simulink library "PTCL_lib"  (Simulink 7.5)
settings: Solver=ode45  StartTime=0.0  StopTime=10.0  RelTol=1e-3
values from neighbouring files (symbols this model uses):
  pPTCL_kw_DeltaTMAvlPwr_TAB = Simulink.Parameter    [PTCL_par.m]
  pPTCL_kw_MaxIDeltaTMAvlPwr_C = Simulink.Parameter    [PTCL_par.m]
  pPTCL_kw_MaxPIDeltaTMAvlPwr_C = Simulink.Parameter    [PTCL_par.m]
  pPTCL_kw_MinIDeltaTMAvlPwr_C = Simulink.Parameter    [PTCL_par.m]
  pPTCL_kw_MinPIDeltaTMAvlPwr_C = Simulink.Parameter    [PTCL_par.m]
  pPTCL_kw_MinTMAvailPwr_C = Simulink.Parameter    [PTCL_par.m]
  pPTCL_kw_PIActDeltaPwrThrsh_C = Simulink.Parameter    [PTCL_par.m]
  pPTCL_kw_PIActHysterDeltaPwr_C = Simulink.Parameter    [PTCL_par.m]
  pPTCL_Nm_MaxTrq_CUR = Simulink.Parameter    [PTCL_par.m]
  pPTCL_Nmps_DrvTrqLowrRateLim_C = Simulink.Parameter    [PTCL_par.m]
  pPTCL_Nmps_DrvTrqUpprRateLim_C = Simulink.Parameter    [PTCL_par.m]
  pPTCL_Nmps_RcpTrqLowrRateLim_C = Simulink.Parameter    [PTCL_par.m]
  pPTCL_Nmps_RcpTrqUpprRateLim_C = Simulink.Parameter    [PTCL_par.m]
  pPTCL_pct_DrvEffiFac_C = Simulink.Parameter    [PTCL_par.m]
  pPTCL_pct_Mot1EffLowrLim_C = Simulink.Parameter    [PTCL_par.m]
  pPTCL_pct_Mot1EffUpprLim_C = Simulink.Parameter    [PTCL_par.m]
  pPTCL_pct_RcpEffiFac_C = Simulink.Parameter    [PTCL_par.m]
  pPTCL_ratio_KI4DeltaTMAvlPwr_CUR = Simulink.Parameter    [PTCL_par.m]
  pPTCL_ratio_KP4DeltaTMAvlPwr_CUR = Simulink.Parameter    [PTCL_par.m]
  pPTCL_ratio_KwToW_M = Simulink.Parameter    [PTCL_par.m]
  pPTCL_ratio_MotSpdFiltFac_C = Simulink.Parameter    [PTCL_par.m]
  pPTCL_ratio_PwrToTrqFac_M = Simulink.Parameter    [PTCL_par.m]
  pPTCL_ratio_WToKw_M = Simulink.Parameter    [PTCL_par.m]
  pPTCL_rpm_RevLowrLim_C = Simulink.Parameter    [PTCL_par.m]
  pPTCL_rpm_RevUpprLim_C = Simulink.Parameter    [PTCL_par.m]
  pPTCL_rpm_TMSpd_TAB = Simulink.Parameter    [PTCL_par.m]
undefined symbols (not defined in the file or in its folder): p_single_Minus_M, p_single_Zero_M, pESPI_kmph_MinSpdSnsrThd_C, pMCI_m_TireDiam_C, pMCI_ratio_KmPerHrToMtrPerSec_C, pMCI_ratio_TrsmRat_C, pMCI_s_NoOfSec_C
libraries: BaseOperationLib_Browser x114, simulink x1
(part 2 of 2)

== system PTCL_lib/PTCL/Algo/MCU1TrqLimCalc/EMSpdFlt ==
  rpm_MCU1TMSpd : Inport
  Abs2 : BaseOperationLib_Browser/Math Operations Changed/Abs  OutMax=[]  OutDataType=fixdt(1, 16)  OutScaling=2^0
  Integrator1 : UnitDelay  SampleTime=-1
      mask Display: patch([0 1 1 1 .75], [1 1 0 .75 1], [0 1 0]);
  LowPassTs : Constant  Value=pPTCL_ratio_MotSpdFiltFac_C
      mask Display: patch([0 1 1 1 .75], [1 1 0 .75 1], [0 1 0]);
  Saturation4 : BaseOperationLib_Browser/Discontinuities Unchanged/Saturation  UpperLimit=14000  LowerLimit=0.5  OutMin=[]  OutMax=[]  OutDataType=fixdt(1, 16)  OutScaling=2^0
      settings: AttributesFormatString=ULim:%<UpperLimit>\nLLim:%<LowerLimit>
  WerghtingFilter : BaseOperationLib_Browser/Discontinuities Unchanged/WerghtingFilter  SystemSampleTime=-1
  rpm_TMSpdFlt : Outport
  wires:
  Saturation4/1 -> rpm_TMSpdFlt/1
  Abs2/1 -> Saturation4/1
  rpm_MCU1TMSpd/1 -> WerghtingFilter/1
  WerghtingFilter/1 -> Abs2/1, Integrator1/1
  Integrator1/1 -> WerghtingFilter/2
  LowPassTs/1 -> WerghtingFilter/3

== system PTCL_lib/PTCL/Algo/MCU2TrqLimCalc/EMSpdFlt ==
  rpm_MCU2TMSpd : Inport
  Abs2 : BaseOperationLib_Browser/Math Operations Changed/Abs  OutMax=[]  OutDataType=fixdt(1, 16)  OutScaling=2^0
  Integrator1 : UnitDelay  SampleTime=-1
      mask Display: patch([0 1 1 1 .75], [1 1 0 .75 1], [0 1 0]);
  LowPassTs : Constant  Value=pPTCL_ratio_MotSpdFiltFac_C
      mask Display: patch([0 1 1 1 .75], [1 1 0 .75 1], [0 1 0]);
  Saturation4 : BaseOperationLib_Browser/Discontinuities Unchanged/Saturation  UpperLimit=14000  LowerLimit=0.5  OutMin=[]  OutMax=[]  OutDataType=fixdt(1, 16)  OutScaling=2^0
      settings: AttributesFormatString=ULim:%<UpperLimit>\nLLim:%<LowerLimit>
  WerghtingFilter : BaseOperationLib_Browser/Discontinuities Unchanged/WerghtingFilter  SystemSampleTime=-1
  rpm_TMSpdFlt : Outport
  wires:
  LowPassTs/1 -> WerghtingFilter/3
  Integrator1/1 -> WerghtingFilter/2
  WerghtingFilter/1 -> Integrator1/1, Abs2/1
  rpm_MCU2TMSpd/1 -> WerghtingFilter/1
  Abs2/1 -> Saturation4/1
  Saturation4/1 -> rpm_TMSpdFlt/1

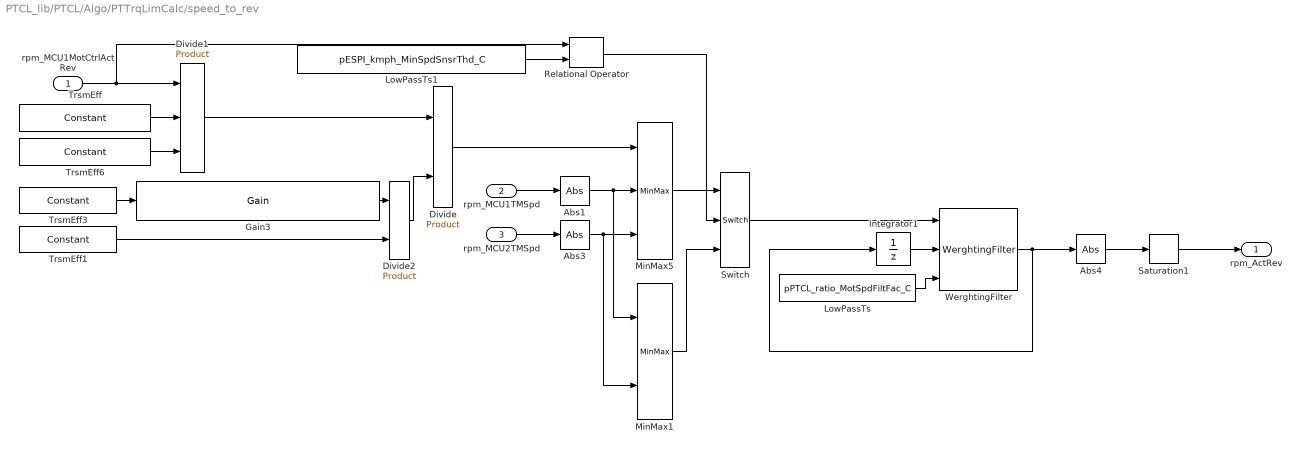
== system PTCL_lib/PTCL/Algo/PTTrqLimCalc/speed_to_rev ==
  rpm_MCU1MotCtrlActRev : Inport
  rpm_MCU1TMSpd : Inport  Port=2
  rpm_MCU2TMSpd : Inport  Port=3
  Abs1 : BaseOperationLib_Browser/Math Operations Changed/Abs  OutMax=[]  OutDataType=fixdt(1, 16)  OutScaling=2^0
  Abs3 : BaseOperationLib_Browser/Math Operations Changed/Abs  OutMax=[]  OutDataType=fixdt(1, 16)  OutScaling=2^0
  Abs4 : BaseOperationLib_Browser/Math Operations Changed/Abs  OutMax=[]  OutDataType=fixdt(1, 16)  OutScaling=2^0
  Divide : BaseOperationLib_Browser/Math Operations Changed/Product  Inputs=*/  Multiplication=Element-wise(.*)  OutMin=[]  OutMax=[]  OutDataType=fixdt(1,16,0)  OutScaling=[]
  Divide1 : BaseOperationLib_Browser/Math Operations Changed/Product  Inputs=***  Multiplication=Element-wise(.*)  OutMin=[]  OutMax=[]  OutDataType=fixdt(1,16,0)  OutScaling=[]
  Divide2 : BaseOperationLib_Browser/Math Operations Changed/Product  Inputs=**  Multiplication=Element-wise(.*)  OutMin=[]  OutMax=[]  OutDataType=fixdt(1,16,0)  OutScaling=[]
  Gain3 : BaseOperationLib_Browser/Math Operations Changed/Gain  Gain=pMCI_ratio_KmPerHrToMtrPerSec_C  Multiplication=Element-wise(K.*u)  ParamMin=[]  ParamMax=[]  ParameterDataType=fixdt(1, 16)  ParameterScalingMode=Best Precision: Matrix-wise  ParameterScaling=2^0  OutMin=[]  OutMax=[]  OutDataType=fixdt(1, 16)  OutScaling=2^0
  Integrator1 : UnitDelay  SampleTime=-1
      mask Display: patch([0 1 1 1 .75], [1 1 0 .75 1], [0 1 0]);
  LowPassTs : Constant  Value=pPTCL_ratio_MotSpdFiltFac_C
      mask Display: patch([0 1 1 1 .75], [1 1 0 .75 1], [0 1 0]);
  LowPassTs1 : Constant  Value=pESPI_kmph_MinSpdSnsrThd_C
      mask Display: patch([0 1 1 1 .75], [1 1 0 .75 1], [0 1 0]);
  MinMax1 : BaseOperationLib_Browser/Math Operations Changed/MinMax  Function=min  Inputs=2  InputSameDT=on  OutMin=[]  OutMax=[]  OutDataType=fixdt(1, 16)  OutScaling=2^0  SaturateOnIntegerOverflow=on
  MinMax5 : BaseOperationLib_Browser/Math Operations Changed/MinMax  Function=min  Inputs=3  InputSameDT=on  OutMin=[]  OutMax=[]  OutDataType=fixdt(1, 16)  OutScaling=2^0  SaturateOnIntegerOverflow=on
  Relational Operator : BaseOperationLib_Browser/Logic Operations Changed/Relational Operator  Operator=>=  InputSameDT=on  LogicOutDataTypeMode=Specify via dialog  LogicDataType=PDT_Bool  OutDataTypeStr=PDT_Bool
  Saturation1 : BaseOperationLib_Browser/Discontinuities Unchanged/Saturation  UpperLimit=pPTCL_rpm_RevUpprLim_C  LowerLimit=pPTCL_rpm_RevLowrLim_C  OutMin=[]  OutMax=[]  OutDataType=fixdt(1, 16)  OutScaling=2^0
      settings: AttributesFormatString=ULim:%<UpperLimit>\nLLim:%<LowerLimit>
  Switch : BaseOperationLib_Browser/Signal Routing Changed/Switch  Criteria=u2 ~= 0  Threshold=1  InputSameDT=on  OutMin=[]  OutMax=[]  OutDataType=fixdt(1,16,0)  OutScaling=[]  SaturateOnIntegerOverflow=on
  TrsmEff : BaseOperationLib_Browser/Sources&Sinks/Constant  Value=pMCI_ratio_TrsmRat_C  OutMin=[]  OutMax=[]  OutDataTypeMode=single  OutDataType=fixdt(1, 16)  ConRadixGroup=Use specified scaling  OutScaling=2^0  OutDataTypeStr=single
  TrsmEff1 : BaseOperationLib_Browser/Sources&Sinks/Constant  Value=pMCI_m_TireDiam_C  OutMin=[]  OutMax=[]  OutDataTypeMode=single  OutDataType=fixdt(1, 16)  ConRadixGroup=Use specified scaling  OutScaling=2^0  OutDataTypeStr=single
  TrsmEff3 : BaseOperationLib_Browser/Sources&Sinks/Constant  Value=pi  OutMin=[]  OutMax=[]  OutDataTypeMode=single  OutDataType=fixdt(1, 16)  ConRadixGroup=Use specified scaling  OutScaling=2^0  OutDataTypeStr=single
  TrsmEff6 : BaseOperationLib_Browser/Sources&Sinks/Constant  Value=pMCI_s_NoOfSec_C  OutMin=[]  OutMax=[]  OutDataTypeMode=single  OutDataType=fixdt(1, 16)  ConRadixGroup=Use specified scaling  OutScaling=2^0  OutDataTypeStr=single
  WerghtingFilter : BaseOperationLib_Browser/Discontinuities Unchanged/WerghtingFilter  SystemSampleTime=-1
  rpm_ActRev : Outport
  wires:
  TrsmEff1/1 -> Divide2/2
  rpm_MCU1MotCtrlActRev/1 -> Divide1/1, Relational Operator/1
  TrsmEff/1 -> Divide1/2
  TrsmEff3/1 -> Gain3/1
  Gain3/1 -> Divide2/1
  Divide1/1 -> Divide/1
  Divide2/1 -> Divide/2
  Switch/1 -> WerghtingFilter/1
  WerghtingFilter/1 -> Integrator1/1, Abs4/1
  Integrator1/1 -> WerghtingFilter/2
  LowPassTs/1 -> WerghtingFilter/3
  Divide/1 -> MinMax5/1
  rpm_MCU1TMSpd/1 -> Abs1/1
  rpm_MCU2TMSpd/1 -> Abs3/1
  MinMax1/1 -> Switch/3
  MinMax5/1 -> Switch/1
  LowPassTs1/1 -> Relational Operator/2
  Relational Operator/1 -> Switch/2
  Abs1/1 -> MinMax5/2, MinMax1/1
  Abs3/1 -> MinMax5/3, MinMax1/2
  Abs4/1 -> Saturation1/1
  Saturation1/1 -> rpm_ActRev/1
  TrsmEff6/1 -> Divide1/3

== system PTCL_lib/PTCL/Algo/CmptPwrLimCalc/BatMaxContiChrgPwrCalc/PwrCtrl ==
  ActPwr : Inport
  TgtPwr : Inport  Port=2
  Enable : EnablePort  StatesWhenEnabling=reset
  Abs1 : Abs  SaturateOnIntegerOverflow=on
      mask Display: patch([0 1 1 1 .75], [1 1 0 .75 1], [0 1 0]);
  Add2 : Sum  SaturateOnIntegerOverflow=on  InputSameDT=on  OutDataTypeStr=Inherit: Same as first input
      mask Display: patch([0 1 1 1 .75], [1 1 0 .75 1], [0 1 0]);
  Add5 : Sum  SaturateOnIntegerOverflow=on  InputSameDT=on  OutDataTypeStr=Inherit: Same as first input
      mask Display: patch([0 1 1 1 .75], [1 1 0 .75 1], [0 1 0]);
  Add6 : Sum  Inputs=+-  SaturateOnIntegerOverflow=on  InputSameDT=on  OutDataTypeStr=Inherit: Same as first input
      mask Display: patch([0 1 1 1 .75], [1 1 0 .75 1], [0 1 0]);
  Constant11 : Constant  Value=pPTCL_kw_MinIDeltaTMAvlPwr_C
      mask Display: patch([0 1 1 1 .75], [1 1 0 .75 1], [0 1 0]);
  Constant12 : Constant  Value=pPTCL_kw_MaxIDeltaTMAvlPwr_C  VectorParams1D=off
      mask Display: patch([0 1 1 1 .75], [1 1 0 .75 1], [0 1 0]);
  Constant13 : Constant  Value=pPTCL_kw_MinPIDeltaTMAvlPwr_C
      mask Display: patch([0 1 1 1 .75], [1 1 0 .75 1], [0 1 0]);
  Constant14 : Constant  Value=pPTCL_kw_MaxPIDeltaTMAvlPwr_C
      mask Display: patch([0 1 1 1 .75], [1 1 0 .75 1], [0 1 0]);
  Constant4 : Constant  Value=p_single_Zero_M
      mask Display: patch([0 1 1 1 .75], [1 1 0 .75 1], [0 1 0]);
  Lookup Table1 : BaseOperationLib_Browser/Lookup Tables Changed/Lookup Table  InputValues=pPTCL_kw_DeltaTMAvlPwr_TAB  Table=pPTCL_ratio_KP4DeltaTMAvlPwr_CUR  LookUpMeth=Interpolation-Use End Values  OutMin=[]  OutMax=[]  OutDataType=fixdt(1, 16)  OutScaling=2^0  OutDataTypeStr=Inherit: Inherit via back propagation  SaturateOnIntegerOverflow=on
      settings: AttributesFormatString=X:%<InputValues>\nTAB:%<Table>
  Lookup Table2 : BaseOperationLib_Browser/Lookup Tables Changed/Lookup Table  InputValues=pPTCL_kw_DeltaTMAvlPwr_TAB  Table=pPTCL_ratio_KI4DeltaTMAvlPwr_CUR  LookUpMeth=Interpolation-Use End Values  OutMin=[]  OutMax=[]  OutDataType=fixdt(1, 16)  OutScaling=2^0  OutDataTypeStr=Inherit: Inherit via back propagation  SaturateOnIntegerOverflow=on
      settings: AttributesFormatString=X:%<InputValues>\nTAB:%<Table>
  MinMax : BaseOperationLib_Browser/Math Operations Changed/MinMax  Function=min  Inputs=2  InputSameDT=on  OutMin=[]  OutMax=[]  OutDataType=fixdt(1,16,0)  OutScaling=[]  SaturateOnIntegerOverflow=on
  Product : BaseOperationLib_Browser/Math Operations Changed/Product  Inputs=2  Multiplication=Element-wise(.*)  OutMin=[]  OutMax=[]  OutDataType=fixdt(1,16,0)  OutScaling=[]  OutDataTypeStr=Inherit: Inherit via back propagation  RndMeth=Zero  SaturateOnIntegerOverflow=on
  Product1 : BaseOperationLib_Browser/Math Operations Changed/Product  Inputs=2  Multiplication=Element-wise(.*)  OutMin=[]  OutMax=[]  OutDataType=fixdt(1,16,0)  OutScaling=[]  OutDataTypeStr=Inherit: Inherit via back propagation  RndMeth=Zero  SaturateOnIntegerOverflow=on
  Saturation Dynamic1 : BaseOperationLib_Browser/Discontinuities Unchanged/Saturation Dynamic  SystemSampleTime=-1  OutMin=[]  OutMax=[]  OutDataTypeStr=Inherit: Same as second input  OutDataType=fixdt(1, 16)  OutScaling=2^-10  DoSatur=on
  Saturation Dynamic2 : BaseOperationLib_Browser/Discontinuities Unchanged/Saturation Dynamic  SystemSampleTime=-1  OutMin=[]  OutMax=[]  OutDataTypeStr=Inherit: Same as second input  OutDataType=fixdt(1, 16)  OutScaling=2^-10  DoSatur=on
  Signal Conversion : SignalConversion  ConversionOutput=Contiguous copy
  Unit Delay2 : BaseOperationLib_Browser/Discrete Unchanged /Unit Delay  X0=0  SampleTime=-1
  DeltaEMAvlPwr : Outport
  wires:
  ActPwr/1 -> Add6/2
  TgtPwr/1 -> Add6/1
  Add6/1 -> Product1/2, Product/2, Lookup Table2/1, Lookup Table1/1
  Add2/1 -> Saturation Dynamic2/2
  Constant14/1 -> Saturation Dynamic2/1
  Constant13/1 -> Saturation Dynamic2/3
  Product1/1 -> Add2/1
  Lookup Table1/1 -> Product1/1
  Product/1 -> Add5/1
  Lookup Table2/1 -> Product/1
  Saturation Dynamic1/1 -> Unit Delay2/1, Add2/2
  Add5/1 -> Saturation Dynamic1/2
  Constant12/1 -> Saturation Dynamic1/1
  Constant11/1 -> Saturation Dynamic1/3
  Unit Delay2/1 -> Add5/2
  Signal Conversion/1 -> DeltaEMAvlPwr/1
  Constant4/1 -> MinMax/1
  Saturation Dynamic2/1 -> MinMax/2
  MinMax/1 -> Abs1/1
  Abs1/1 -> Signal Conversion/1

== system PTCL_lib/PTCL/Algo/CmptPwrLimCalc/BatMaxContiDschPwrCalc/PwrCtrl ==
  ActPwr : Inport
  TgtPwr : Inport  Port=2
  Enable : EnablePort  StatesWhenEnabling=reset
  Abs1 : Abs  SaturateOnIntegerOverflow=on
      mask Display: patch([0 1 1 1 .75], [1 1 0 .75 1], [0 1 0]);
  Add2 : Sum  SaturateOnIntegerOverflow=on  InputSameDT=on  OutDataTypeStr=Inherit: Same as first input
      mask Display: patch([0 1 1 1 .75], [1 1 0 .75 1], [0 1 0]);
  Add5 : Sum  SaturateOnIntegerOverflow=on  InputSameDT=on  OutDataTypeStr=Inherit: Same as first input
      mask Display: patch([0 1 1 1 .75], [1 1 0 .75 1], [0 1 0]);
  Add6 : Sum  Inputs=+-  SaturateOnIntegerOverflow=on  InputSameDT=on  OutDataTypeStr=Inherit: Same as first input
      mask Display: patch([0 1 1 1 .75], [1 1 0 .75 1], [0 1 0]);
  Constant11 : Constant  Value=pPTCL_kw_MinIDeltaTMAvlPwr_C
      mask Display: patch([0 1 1 1 .75], [1 1 0 .75 1], [0 1 0]);
  Constant12 : Constant  Value=pPTCL_kw_MaxIDeltaTMAvlPwr_C  VectorParams1D=off
      mask Display: patch([0 1 1 1 .75], [1 1 0 .75 1], [0 1 0]);
  Constant13 : Constant  Value=pPTCL_kw_MinPIDeltaTMAvlPwr_C
      mask Display: patch([0 1 1 1 .75], [1 1 0 .75 1], [0 1 0]);
  Constant14 : Constant  Value=pPTCL_kw_MaxPIDeltaTMAvlPwr_C
      mask Display: patch([0 1 1 1 .75], [1 1 0 .75 1], [0 1 0]);
  Constant4 : Constant  Value=p_single_Zero_M
      mask Display: patch([0 1 1 1 .75], [1 1 0 .75 1], [0 1 0]);
  Lookup Table1 : BaseOperationLib_Browser/Lookup Tables Changed/Lookup Table  InputValues=pPTCL_kw_DeltaTMAvlPwr_TAB  Table=pPTCL_ratio_KP4DeltaTMAvlPwr_CUR  LookUpMeth=Interpolation-Use End Values  OutMin=[]  OutMax=[]  OutDataType=fixdt(1, 16)  OutScaling=2^0  OutDataTypeStr=Inherit: Inherit via back propagation  SaturateOnIntegerOverflow=on
      settings: AttributesFormatString=X:%<InputValues>\nTAB:%<Table>
  Lookup Table2 : BaseOperationLib_Browser/Lookup Tables Changed/Lookup Table  InputValues=pPTCL_kw_DeltaTMAvlPwr_TAB  Table=pPTCL_ratio_KI4DeltaTMAvlPwr_CUR  LookUpMeth=Interpolation-Use End Values  OutMin=[]  OutMax=[]  OutDataType=fixdt(1, 16)  OutScaling=2^0  OutDataTypeStr=Inherit: Inherit via back propagation  SaturateOnIntegerOverflow=on
      settings: AttributesFormatString=X:%<InputValues>\nTAB:%<Table>
  MinMax : BaseOperationLib_Browser/Math Operations Changed/MinMax  Function=min  Inputs=2  InputSameDT=on  OutMin=[]  OutMax=[]  OutDataType=fixdt(1,16,0)  OutScaling=[]  SaturateOnIntegerOverflow=on
  Product : BaseOperationLib_Browser/Math Operations Changed/Product  Inputs=2  Multiplication=Element-wise(.*)  OutMin=[]  OutMax=[]  OutDataType=fixdt(1,16,0)  OutScaling=[]  OutDataTypeStr=Inherit: Inherit via back propagation  RndMeth=Zero  SaturateOnIntegerOverflow=on
  Product1 : BaseOperationLib_Browser/Math Operations Changed/Product  Inputs=2  Multiplication=Element-wise(.*)  OutMin=[]  OutMax=[]  OutDataType=fixdt(1,16,0)  OutScaling=[]  OutDataTypeStr=Inherit: Inherit via back propagation  RndMeth=Zero  SaturateOnIntegerOverflow=on
  Saturation Dynamic1 : BaseOperationLib_Browser/Discontinuities Unchanged/Saturation Dynamic  SystemSampleTime=-1  OutMin=[]  OutMax=[]  OutDataTypeStr=Inherit: Same as second input  OutDataType=fixdt(1, 16)  OutScaling=2^-10  DoSatur=on
  Saturation Dynamic2 : BaseOperationLib_Browser/Discontinuities Unchanged/Saturation Dynamic  SystemSampleTime=-1  OutMin=[]  OutMax=[]  OutDataTypeStr=Inherit: Same as second input  OutDataType=fixdt(1, 16)  OutScaling=2^-10  DoSatur=on
  Signal Conversion : SignalConversion  ConversionOutput=Contiguous copy
  Unit Delay2 : BaseOperationLib_Browser/Discrete Unchanged /Unit Delay  X0=0  SampleTime=-1
  DeltaEMAvlPwr : Outport
  wires:
  ActPwr/1 -> Add6/2
  TgtPwr/1 -> Add6/1
  Add6/1 -> Product1/2, Product/2, Lookup Table2/1, Lookup Table1/1
  Add2/1 -> Saturation Dynamic2/2
  Constant14/1 -> Saturation Dynamic2/1
  Constant13/1 -> Saturation Dynamic2/3
  Product1/1 -> Add2/1
  Lookup Table1/1 -> Product1/1
  Product/1 -> Add5/1
  Lookup Table2/1 -> Product/1
  Saturation Dynamic1/1 -> Unit Delay2/1, Add2/2
  Add5/1 -> Saturation Dynamic1/2
  Constant12/1 -> Saturation Dynamic1/1
  Constant11/1 -> Saturation Dynamic1/3
  Unit Delay2/1 -> Add5/2
  Signal Conversion/1 -> DeltaEMAvlPwr/1
  Constant4/1 -> MinMax/1
  Saturation Dynamic2/1 -> MinMax/2
  MinMax/1 -> Abs1/1
  Abs1/1 -> Signal Conversion/1

== system PTCL_lib/PTCL/Algo/CmptPwrLimCalc/BatMaxPeakChrgPwrCalc/PwrCtrl ==
  ActPwr : Inport
  TgtPwr : Inport  Port=2
  Enable : EnablePort  StatesWhenEnabling=reset
  Abs1 : Abs  SaturateOnIntegerOverflow=on
      mask Display: patch([0 1 1 1 .75], [1 1 0 .75 1], [0 1 0]);
  Add2 : Sum  SaturateOnIntegerOverflow=on  InputSameDT=on  OutDataTypeStr=Inherit: Same as first input
      mask Display: patch([0 1 1 1 .75], [1 1 0 .75 1], [0 1 0]);
  Add5 : Sum  SaturateOnIntegerOverflow=on  InputSameDT=on  OutDataTypeStr=Inherit: Same as first input
      mask Display: patch([0 1 1 1 .75], [1 1 0 .75 1], [0 1 0]);
  Add6 : Sum  Inputs=+-  SaturateOnIntegerOverflow=on  InputSameDT=on  OutDataTypeStr=Inherit: Same as first input
      mask Display: patch([0 1 1 1 .75], [1 1 0 .75 1], [0 1 0]);
  Constant11 : Constant  Value=pPTCL_kw_MinIDeltaTMAvlPwr_C
      mask Display: patch([0 1 1 1 .75], [1 1 0 .75 1], [0 1 0]);
  Constant12 : Constant  Value=pPTCL_kw_MaxIDeltaTMAvlPwr_C  VectorParams1D=off
      mask Display: patch([0 1 1 1 .75], [1 1 0 .75 1], [0 1 0]);
  Constant13 : Constant  Value=pPTCL_kw_MinPIDeltaTMAvlPwr_C
      mask Display: patch([0 1 1 1 .75], [1 1 0 .75 1], [0 1 0]);
  Constant14 : Constant  Value=pPTCL_kw_MaxPIDeltaTMAvlPwr_C
      mask Display: patch([0 1 1 1 .75], [1 1 0 .75 1], [0 1 0]);
  Constant4 : Constant  Value=p_single_Zero_M
      mask Display: patch([0 1 1 1 .75], [1 1 0 .75 1], [0 1 0]);
  Lookup Table1 : BaseOperationLib_Browser/Lookup Tables Changed/Lookup Table  InputValues=pPTCL_kw_DeltaTMAvlPwr_TAB  Table=pPTCL_ratio_KP4DeltaTMAvlPwr_CUR  LookUpMeth=Interpolation-Use End Values  OutMin=[]  OutMax=[]  OutDataType=fixdt(1, 16)  OutScaling=2^0  OutDataTypeStr=Inherit: Inherit via back propagation  SaturateOnIntegerOverflow=on
      settings: AttributesFormatString=X:%<InputValues>\nTAB:%<Table>
  Lookup Table2 : BaseOperationLib_Browser/Lookup Tables Changed/Lookup Table  InputValues=pPTCL_kw_DeltaTMAvlPwr_TAB  Table=pPTCL_ratio_KI4DeltaTMAvlPwr_CUR  LookUpMeth=Interpolation-Use End Values  OutMin=[]  OutMax=[]  OutDataType=fixdt(1, 16)  OutScaling=2^0  OutDataTypeStr=Inherit: Inherit via back propagation  SaturateOnIntegerOverflow=on
      settings: AttributesFormatString=X:%<InputValues>\nTAB:%<Table>
  MinMax : BaseOperationLib_Browser/Math Operations Changed/MinMax  Function=min  Inputs=2  InputSameDT=on  OutMin=[]  OutMax=[]  OutDataType=fixdt(1,16,0)  OutScaling=[]  SaturateOnIntegerOverflow=on
  Product : BaseOperationLib_Browser/Math Operations Changed/Product  Inputs=2  Multiplication=Element-wise(.*)  OutMin=[]  OutMax=[]  OutDataType=fixdt(1,16,0)  OutScaling=[]  OutDataTypeStr=Inherit: Inherit via back propagation  RndMeth=Zero  SaturateOnIntegerOverflow=on
  Product1 : BaseOperationLib_Browser/Math Operations Changed/Product  Inputs=2  Multiplication=Element-wise(.*)  OutMin=[]  OutMax=[]  OutDataType=fixdt(1,16,0)  OutScaling=[]  OutDataTypeStr=Inherit: Inherit via back propagation  RndMeth=Zero  SaturateOnIntegerOverflow=on
  Saturation Dynamic1 : BaseOperationLib_Browser/Discontinuities Unchanged/Saturation Dynamic  SystemSampleTime=-1  OutMin=[]  OutMax=[]  OutDataTypeStr=Inherit: Same as second input  OutDataType=fixdt(1, 16)  OutScaling=2^-10  DoSatur=on
  Saturation Dynamic2 : BaseOperationLib_Browser/Discontinuities Unchanged/Saturation Dynamic  SystemSampleTime=-1  OutMin=[]  OutMax=[]  OutDataTypeStr=Inherit: Same as second input  OutDataType=fixdt(1, 16)  OutScaling=2^-10  DoSatur=on
  Signal Conversion : SignalConversion  ConversionOutput=Contiguous copy
  Unit Delay2 : BaseOperationLib_Browser/Discrete Unchanged /Unit Delay  X0=0  SampleTime=-1
  DeltaEMAvlPwr : Outport
  wires:
  ActPwr/1 -> Add6/2
  TgtPwr/1 -> Add6/1
  Add6/1 -> Product1/2, Product/2, Lookup Table2/1, Lookup Table1/1
  Add2/1 -> Saturation Dynamic2/2
  Constant14/1 -> Saturation Dynamic2/1
  Constant13/1 -> Saturation Dynamic2/3
  Product1/1 -> Add2/1
  Lookup Table1/1 -> Product1/1
  Product/1 -> Add5/1
  Lookup Table2/1 -> Product/1
  Saturation Dynamic1/1 -> Unit Delay2/1, Add2/2
  Add5/1 -> Saturation Dynamic1/2
  Constant12/1 -> Saturation Dynamic1/1
  Constant11/1 -> Saturation Dynamic1/3
  Unit Delay2/1 -> Add5/2
  Signal Conversion/1 -> DeltaEMAvlPwr/1
  Constant4/1 -> MinMax/1
  Saturation Dynamic2/1 -> MinMax/2
  MinMax/1 -> Abs1/1
  Abs1/1 -> Signal Conversion/1

== system PTCL_lib/PTCL/Algo/CmptPwrLimCalc/BatMaxPeakDschPwrCalc/PwrCtrl ==
  ActPwr : Inport
  TgtPwr : Inport  Port=2
  Enable : EnablePort  StatesWhenEnabling=reset
  Abs1 : Abs  SaturateOnIntegerOverflow=on
      mask Display: patch([0 1 1 1 .75], [1 1 0 .75 1], [0 1 0]);
  Add2 : Sum  SaturateOnIntegerOverflow=on  InputSameDT=on  OutDataTypeStr=Inherit: Same as first input
      mask Display: patch([0 1 1 1 .75], [1 1 0 .75 1], [0 1 0]);
  Add5 : Sum  SaturateOnIntegerOverflow=on  InputSameDT=on  OutDataTypeStr=Inherit: Same as first input
      mask Display: patch([0 1 1 1 .75], [1 1 0 .75 1], [0 1 0]);
  Add6 : Sum  Inputs=+-  SaturateOnIntegerOverflow=on  InputSameDT=on  OutDataTypeStr=Inherit: Same as first input
      mask Display: patch([0 1 1 1 .75], [1 1 0 .75 1], [0 1 0]);
  Constant11 : Constant  Value=pPTCL_kw_MinIDeltaTMAvlPwr_C
      mask Display: patch([0 1 1 1 .75], [1 1 0 .75 1], [0 1 0]);
  Constant12 : Constant  Value=pPTCL_kw_MaxIDeltaTMAvlPwr_C  VectorParams1D=off
      mask Display: patch([0 1 1 1 .75], [1 1 0 .75 1], [0 1 0]);
  Constant13 : Constant  Value=pPTCL_kw_MinPIDeltaTMAvlPwr_C
      mask Display: patch([0 1 1 1 .75], [1 1 0 .75 1], [0 1 0]);
  Constant14 : Constant  Value=pPTCL_kw_MaxPIDeltaTMAvlPwr_C
      mask Display: patch([0 1 1 1 .75], [1 1 0 .75 1], [0 1 0]);
  Constant4 : Constant  Value=p_single_Zero_M
      mask Display: patch([0 1 1 1 .75], [1 1 0 .75 1], [0 1 0]);
  Lookup Table1 : BaseOperationLib_Browser/Lookup Tables Changed/Lookup Table  InputValues=pPTCL_kw_DeltaTMAvlPwr_TAB  Table=pPTCL_ratio_KP4DeltaTMAvlPwr_CUR  LookUpMeth=Interpolation-Use End Values  OutMin=[]  OutMax=[]  OutDataType=fixdt(1, 16)  OutScaling=2^0  OutDataTypeStr=Inherit: Inherit via back propagation  SaturateOnIntegerOverflow=on
      settings: AttributesFormatString=X:%<InputValues>\nTAB:%<Table>
  Lookup Table2 : BaseOperationLib_Browser/Lookup Tables Changed/Lookup Table  InputValues=pPTCL_kw_DeltaTMAvlPwr_TAB  Table=pPTCL_ratio_KI4DeltaTMAvlPwr_CUR  LookUpMeth=Interpolation-Use End Values  OutMin=[]  OutMax=[]  OutDataType=fixdt(1, 16)  OutScaling=2^0  OutDataTypeStr=Inherit: Inherit via back propagation  SaturateOnIntegerOverflow=on
      settings: AttributesFormatString=X:%<InputValues>\nTAB:%<Table>
  MinMax : BaseOperationLib_Browser/Math Operations Changed/MinMax  Function=min  Inputs=2  InputSameDT=on  OutMin=[]  OutMax=[]  OutDataType=fixdt(1,16,0)  OutScaling=[]  SaturateOnIntegerOverflow=on
  Product : BaseOperationLib_Browser/Math Operations Changed/Product  Inputs=2  Multiplication=Element-wise(.*)  OutMin=[]  OutMax=[]  OutDataType=fixdt(1,16,0)  OutScaling=[]  OutDataTypeStr=Inherit: Inherit via back propagation  RndMeth=Zero  SaturateOnIntegerOverflow=on
  Product1 : BaseOperationLib_Browser/Math Operations Changed/Product  Inputs=2  Multiplication=Element-wise(.*)  OutMin=[]  OutMax=[]  OutDataType=fixdt(1,16,0)  OutScaling=[]  OutDataTypeStr=Inherit: Inherit via back propagation  RndMeth=Zero  SaturateOnIntegerOverflow=on
  Saturation Dynamic1 : BaseOperationLib_Browser/Discontinuities Unchanged/Saturation Dynamic  SystemSampleTime=-1  OutMin=[]  OutMax=[]  OutDataTypeStr=Inherit: Same as second input  OutDataType=fixdt(1, 16)  OutScaling=2^-10  DoSatur=on
  Saturation Dynamic2 : BaseOperationLib_Browser/Discontinuities Unchanged/Saturation Dynamic  SystemSampleTime=-1  OutMin=[]  OutMax=[]  OutDataTypeStr=Inherit: Same as second input  OutDataType=fixdt(1, 16)  OutScaling=2^-10  DoSatur=on
  Signal Conversion : SignalConversion  ConversionOutput=Contiguous copy
  Unit Delay2 : BaseOperationLib_Browser/Discrete Unchanged /Unit Delay  X0=0  SampleTime=-1
  DeltaEMAvlPwr : Outport
  wires:
  ActPwr/1 -> Add6/2
  TgtPwr/1 -> Add6/1
  Add6/1 -> Product1/2, Product/2, Lookup Table2/1, Lookup Table1/1
  Add2/1 -> Saturation Dynamic2/2
  Constant14/1 -> Saturation Dynamic2/1
  Constant13/1 -> Saturation Dynamic2/3
  Product1/1 -> Add2/1
  Lookup Table1/1 -> Product1/1
  Product/1 -> Add5/1
  Lookup Table2/1 -> Product/1
  Saturation Dynamic1/1 -> Unit Delay2/1, Add2/2
  Add5/1 -> Saturation Dynamic1/2
  Constant12/1 -> Saturation Dynamic1/1
  Constant11/1 -> Saturation Dynamic1/3
  Unit Delay2/1 -> Add5/2
  Signal Conversion/1 -> DeltaEMAvlPwr/1
  Constant4/1 -> MinMax/1
  Saturation Dynamic2/1 -> MinMax/2
  MinMax/1 -> Abs1/1
  Abs1/1 -> Signal Conversion/1
